simulink model "lqr_control"  (R2020b)
settings: Solver=VariableStepAuto  StartTime=0.0  StopTime=100  RelTol=1e-3
values from neighbouring files (symbols this model uses):
  A_m = [0 1 0 ... (first row only)    [autopilot.m]
  B_m = [0; M_delta; Tc/m]    [autopilot.m]
  C_m = diag([1 1 1])    [autopilot.m]
  D_m = [0;0;0]    [autopilot.m]
  K_1 = K(1)    [autopilot.m]
  K_2 = K(2)    [autopilot.m]
  K_3 = K(3)    [autopilot.m]
undefined symbols (not defined in the file or in its folder): Earth, WGS84
libraries: aerolibtransform2 x1, aerolibfltsims x1
settings Model: Creator=shohei  LastModifiedBy=shohei

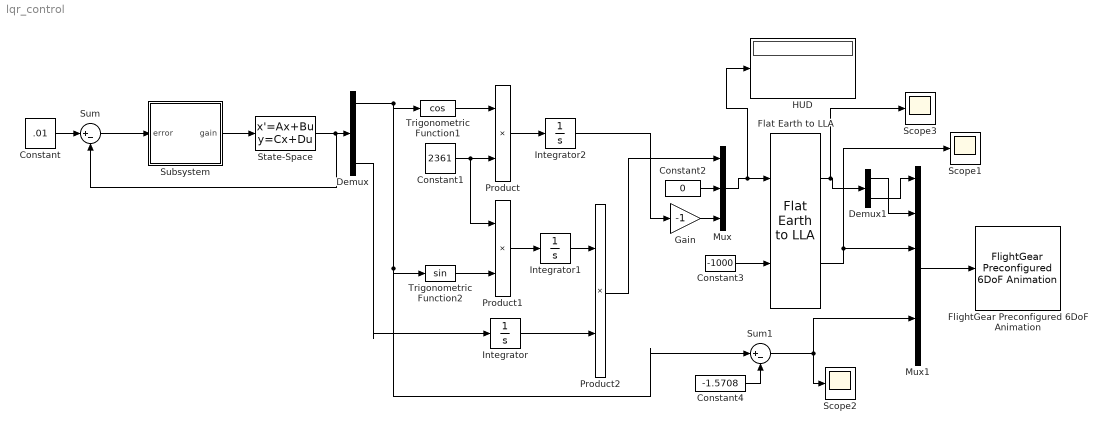
== system lqr_control ==
  Constant : Constant  Value=.01
  Constant1 : Constant  Value=2361
  Constant2 : Constant  Value=0
  Constant3 : Constant  Value=-1000
  Constant4 : Constant  Value=-1.5708
  Demux : Demux  Outputs=3
  Demux1 : Demux  Outputs=2
  Flat Earth to LLA : aerolibtransform2/Flat Earth to LLA  units=Metric (MKS)  ptype=Earth (WGS84)  F=1/298.257223563  R=6378137  refPosPort=off  LL0=[0 10]  psi=0
  FlightGear Preconfigured 6DoF Animation : aerolibfltsims/FlightGear Preconfigured 6DoF Animation  xFlightGearVersion=v2019.1  DestinationIpAddress=127.0.0.1  DestinationPort=5502  SampleTime=1/30  packetVersion=24
  Gain : Gain  Gain=-1
  HUD : Display
  Integrator : Integrator
  Integrator1 : Integrator
  Integrator2 : Integrator
  Mux : Mux  Inputs=3
  Mux1 : Mux  Inputs=6
  Product : Product
  Product1 : Product
  Product2 : Product
  Scope1 : Scope
  Scope2 : Scope
  Scope3 : Scope
  State-Space : StateSpace  A=A_m  B=B_m  C=C_m  D=D_m  InitialCondition=[0.2;0;0]
  Subsystem : Subsystem
  Sum : Sum  Inputs=|+-
  Sum1 : Sum  Inputs=|+-
  Trigonometric Function1 : Trigonometry  Operator=cos
  Trigonometric Function2 : Trigonometry
  wires:
  Constant/1 -> Sum/1
  Sum/1 -> Subsystem/1(error)
  Subsystem/1(gain) -> State-Space/1
  State-Space/1 -> Sum/2, Demux/1
  Demux/1 -> Sum1/1, Trigonometric Function2/1, Trigonometric Function1/1
  Trigonometric Function1/1 -> Product/1
  Constant1/1 -> Product1/1, Product/2
  Trigonometric Function2/1 -> Product1/2
  Demux/3 -> Integrator/1
  Product1/1 -> Integrator1/1
  Integrator1/1 -> Product2/1
  Integrator/1 -> Product2/2
  Product/1 -> Integrator2/1
  Gain/1 -> Mux/3
  Integrator2/1 -> Gain/1
  Product2/1 -> Mux/1
  Constant2/1 -> Mux/2
  Mux/1 -> HUD/1, Flat Earth to LLA/1
  Constant3/1 -> Flat Earth to LLA/2
  Flat Earth to LLA/1 -> Scope3/1, Demux1/1
  Demux1/1 -> Mux1/2
  Demux1/2 -> Mux1/1
  Flat Earth to LLA/2 -> Mux1/3, Scope1/1
  Constant4/1 -> Sum1/2
  Sum1/1 -> Mux1/5, Scope2/1
  Mux1/1 -> FlightGear Preconfigured 6DoF Animation/1

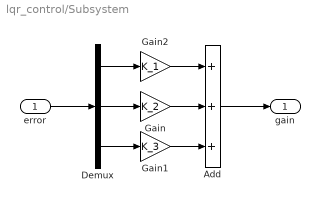
== system lqr_control/Subsystem ==
  error : Inport
  Add : Sum  Inputs=+++
  Demux : Demux  Outputs=3
  Gain : Gain  Gain=K_2
  Gain1 : Gain  Gain=K_3
  Gain2 : Gain  Gain=K_1
  gain : Outport
  wires:
  error/1 -> Demux/1
  Gain2/1 -> Add/1
  Add/1 -> gain/1
  Gain1/1 -> Add/3
  Demux/2 -> Gain/1
  Demux/3 -> Gain1/1
  Gain/1 -> Add/2
  Demux/1 -> Gain2/1
